simulink model "simscape_basic"  (R2024b)
settings: Solver=VariableStepAuto  StartTime=0.0  StopTime=inf  FixedStep=timestep  RelTol=1e-6
values from neighbouring files (symbols this model uses):
  timestep = 0.5    [design_details.m]
libraries: aircraft_refuel_control x1, simulink x1, GS_refuel_control x1
settings Model: PacingRate=5  Creator=MW  LastModifiedBy=MW
settings SolverCC: MaxConsecutiveMinStep=3
settings ModelReferenceCC: UpdateModelReferenceTargets=IfOutOfDate
settings SFSimCC: SimTargetLang=C++

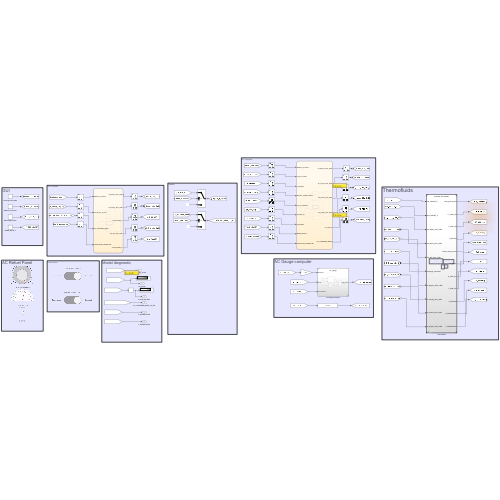
[thumbnail: Simulink's stored preview of the top-level diagram]
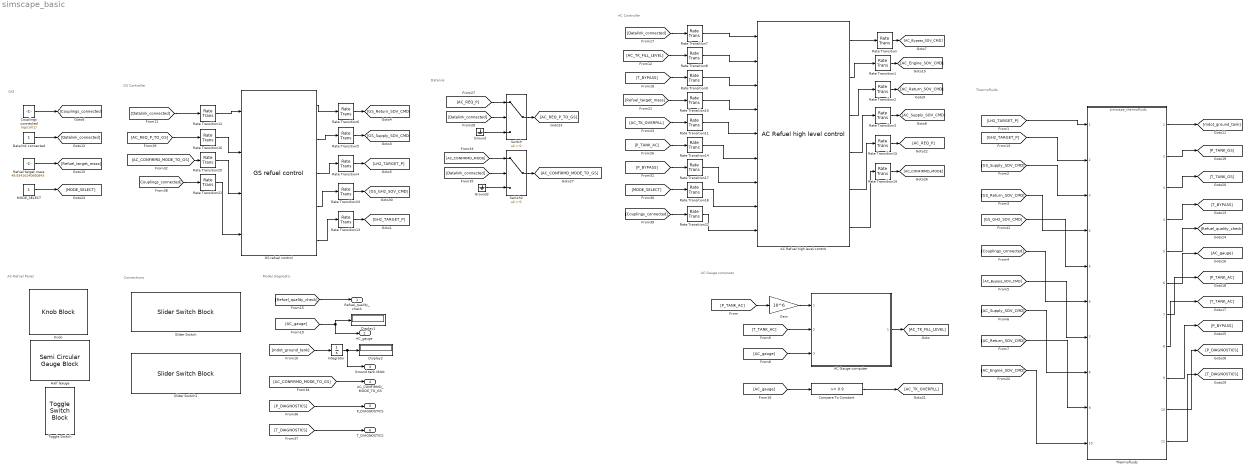
== system simscape_basic ==
  note: Thermofluids
  note: AC Refuel Panel
  note: GUI
  note: Model diagnostic
  note: Connections
  note: GS Controller
  note: AC Controller
  note: AC Gauge computer
  note: Datalink
  AC Gauge computer : Subsystem  ReferencedSubsystem=AC_gauge
  AC Refuel high level control : aircraft_refuel_control/AC Refuel high level control  SystemSampleTime=timestep  VariantActivationTime=update diagram  AllowFlexibleInterface=on  Latency=0  AutoFrameSizeCalculation=off
  Compare To Constant : simulink/Logic and Bit Operations/Compare To Constant  relop=>=  const=0.9  OutDataTypeStr=boolean
  Couplings connected : Constant  Value=logical(1)
  Datalink connected : Constant
  Display1 : Display
  Display2 : Display
  GS refuel control : GS_refuel_control/GS refuel control  SystemSampleTime=timestep  VariantActivationTime=update diagram  AllowFlexibleInterface=on  Latency=0  AutoFrameSizeCalculation=off
  Gain : Gain  Gain=10^6
  Ground : Ground
  Ground2 : Ground
  Half Gauge : SemiCircularGaugeBlock  ScaleMax=28
  Integrator : Integrator
  Knob : KnobBlock  ScaleMax=28
  MODE_SELECT : Constant
  Rate Transition{,1..23} (24 alike) : RateTransition
  Refuel target mass : Constant  Value=48.83416240660843
  Slider Switch : SliderSwitchBlock
      settings: Values={{'Disconnected', 'Connected'}, [0 1]}
  Slider Switch1 : SliderSwitchBlock
      settings: Values={{'Disconnected', 'Connected'}, [0 1]}
  Switch : Switch  Criteria=u2 > Threshold  SaturateOnIntegerOverflow=off  InputSameDT=off
  Switch2 : Switch  Criteria=u2 > Threshold  SaturateOnIntegerOverflow=off  InputSameDT=off
  Thermofluids : ModelReference  ModelNameDialog=simscape_thermofluids.slx  SimulationMode=Normal  ModelReferenceVersion=1.172
  Toggle Switch : ToggleSwitchBlock
      settings: Values={{'DEFUEL', 'REFUEL'}, [0 1]}
  Refuel_quality_check : Outport
  AC_gauge : Outport  Port=2
  Ground tank Mdot : Outport  Port=3
  AC_CONFIRMD_MODE_TO_GS : Outport  Port=4
  P_DIAGNOSTICS : Outport  Port=5
  T_DIAGNOSTICS : Outport  Port=6
  wires:
  Couplings connected/1 -> [Couplings_connected]
  [AC_TK_FILL_LEVEL] -> Rate Transition8/1
  [mdot_ground_tank] -> Integrator/1
  Integrator/1 -> Ground tank Mdot/1, Display2/1
  Datalink connected/1 -> [Datalink_connected]
  [Datalink_connected] -> Rate Transition7/1
  [Datalink_connected] -> Rate Transition12/1
  AC Refuel high level control/1 -> Rate Transition/1
  AC Refuel high level control/2 -> Rate Transition1/1
  [T_BYPASS] -> Rate Transition9/1
  GS refuel control/1 -> Rate Transition6/1
  [Refuel_quality_check] -> Refuel_quality_check/1
  [AC_gauge] -> Display1/1, AC_gauge/1
  Refuel target mass/1 -> [Refuel_target_mass]
  [LH2_TARGET_P] -> Thermofluids/1
  Rate Transition2/1 -> [AC_Return_SOV_CMD]
  Rate Transition3/1 -> [AC_Supply_SOV_CMD]
  Rate Transition4/1 -> [LH2_TARGET_P]
  AC Refuel high level control/4 -> Rate Transition3/1
  AC Refuel high level control/3 -> Rate Transition2/1
  Rate Transition1/1 -> [AC_Engine_SOV_CMD]
  Rate Transition/1 -> [AC_Bypass_SOV_CMD]
  GS refuel control/2 -> Rate Transition5/1
  Rate Transition5/1 -> [GS_Supply_SOV_CMD]
  Rate Transition6/1 -> [GS_Return_SOV_CMD]
  [AC_gauge] -> AC Gauge computer/3
  AC Gauge computer/1 -> [AC_TK_FILL_LEVEL]
  [P_TANK_AC] -> Gain/1
  [T_TANK_AC] -> AC Gauge computer/2
  Gain/1 -> AC Gauge computer/1
  [Refuel_target_mass] -> Rate Transition10/1
  [AC_gauge] -> Compare To Constant/1
  Compare To Constant/1 -> [AC_TK_OVERFILL]
  [AC_TK_OVERFILL] -> Rate Transition11/1
  Rate Transition12/1 -> GS refuel control/1
  Rate Transition11/1 -> AC Refuel high level control/5
  [P_TANK_AC] -> Rate Transition14/1
  Rate Transition14/1 -> AC Refuel high level control/6
  AC Refuel high level control/5 -> Rate Transition15/1
  Rate Transition15/1 -> [AC_REQ_P]
  [AC_REQ_P] -> Switch/1
  [Datalink_connected] -> Switch/2
  Ground/1 -> Switch/3
  Switch/1 -> [AC_REQ_P_TO_GS]
  [AC_REQ_P_TO_GS] -> Rate Transition16/1
  MODE_SELECT/1 -> [MODE_SELECT]
  GS refuel control/3 -> Rate Transition4/1
  [P_BYPASS] -> Rate Transition17/1
  [MODE_SELECT] -> Rate Transition18/1
  Rate Transition17/1 -> AC Refuel high level control/7
  Rate Transition18/1 -> AC Refuel high level control/8
  Rate Transition19/1 -> [AC_CONFIRMD_MODE]
  AC Refuel high level control/6 -> Rate Transition19/1
  [AC_CONFIRMD_MODE] -> Switch2/1
  [Datalink_connected] -> Switch2/2
  Ground2/1 -> Switch2/3
  Switch2/1 -> [AC_CONFIRMD_MODE_TO_GS]
  [AC_CONFIRMD_MODE_TO_GS] -> Rate Transition20/1
  [AC_CONFIRMD_MODE_TO_GS] -> AC_CONFIRMD_MODE_TO_GS/1
  [P_DIAGNOSTICS] -> P_DIAGNOSTICS/1
  [T_DIAGNOSTICS] -> T_DIAGNOSTICS/1
  [Couplings_connected] -> Rate Transition21/1
  [Couplings_connected] -> Rate Transition22/1
  Rate Transition22/1 -> AC Refuel high level control/9
  Rate Transition23/1 -> [GS_GH2_SOV_CMD]
  GS refuel control/4 -> Rate Transition23/1
  Rate Transition10/1 -> AC Refuel high level control/4
  Rate Transition9/1 -> AC Refuel high level control/3
  Rate Transition8/1 -> AC Refuel high level control/2
  Rate Transition7/1 -> AC Refuel high level control/1
  Rate Transition16/1 -> GS refuel control/2
  Rate Transition20/1 -> GS refuel control/3
  Rate Transition21/1 -> GS refuel control/4
  Thermofluids/1 -> [mdot_ground_tank]
  Thermofluids/2 -> [P_TANK_GS]
  Thermofluids/3 -> [T_TANK_GS]
  Thermofluids/4 -> [T_BYPASS]
  Thermofluids/5 -> [Refuel_quality_check]
  Thermofluids/6 -> [AC_gauge]
  Thermofluids/7 -> [P_TANK_AC]
  Thermofluids/8 -> [T_TANK_AC]
  Thermofluids/9 -> [P_BYPASS]
  Thermofluids/10 -> [P_DIAGNOSTICS]
  Thermofluids/11 -> [T_DIAGNOSTICS]
  Rate Transition13/1 -> [GH2_TARGET_P]
  GS refuel control/5 -> Rate Transition13/1
  [GH2_TARGET_P] -> Thermofluids/2
  [GS_Supply_SOV_CMD] -> Thermofluids/3
  [GS_Return_SOV_CMD] -> Thermofluids/4
  [GS_GH2_SOV_CMD] -> Thermofluids/5
  [Couplings_connected] -> Thermofluids/6
  [AC_Bypass_SOV_CMD] -> Thermofluids/7
  [AC_Supply_SOV_CMD] -> Thermofluids/8
  [AC_Return_SOV_CMD] -> Thermofluids/9
  [AC_Engine_SOV_CMD] -> Thermofluids/10
